simulink model "bnbRL_Plant"  (R2026a)
settings: Solver=VariableStepAuto
values from neighbouring files (symbols this model uses):
  d = 0.016    [bnbInit.m]    (also in bnbRL_Animation.m)
  g = 9.81    [bnbInit.m]
  K_BB = (R^2 * m * g * d) / (L * (m * R^2 + J))    (= 0.424676496462)    [bnbInit.m]
  L = 0.264    [bnbInit.m]    (also in bnbRL_Animation.m)
  x0 = 0    [bnbInit.m]
  xdot0 = 0    [bnbInit.m]
settings Model: Creator=user  LastModifiedBy=user

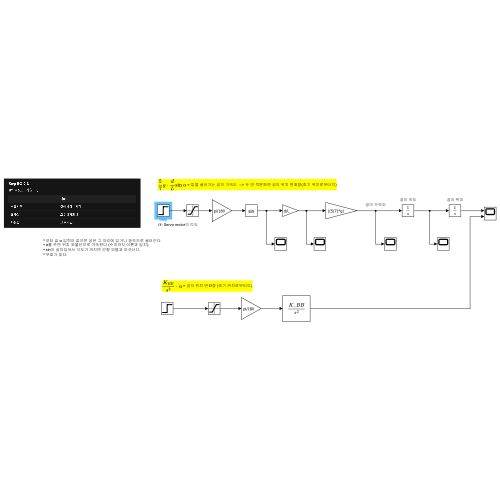
[thumbnail: Simulink's stored preview of the top-level diagram]
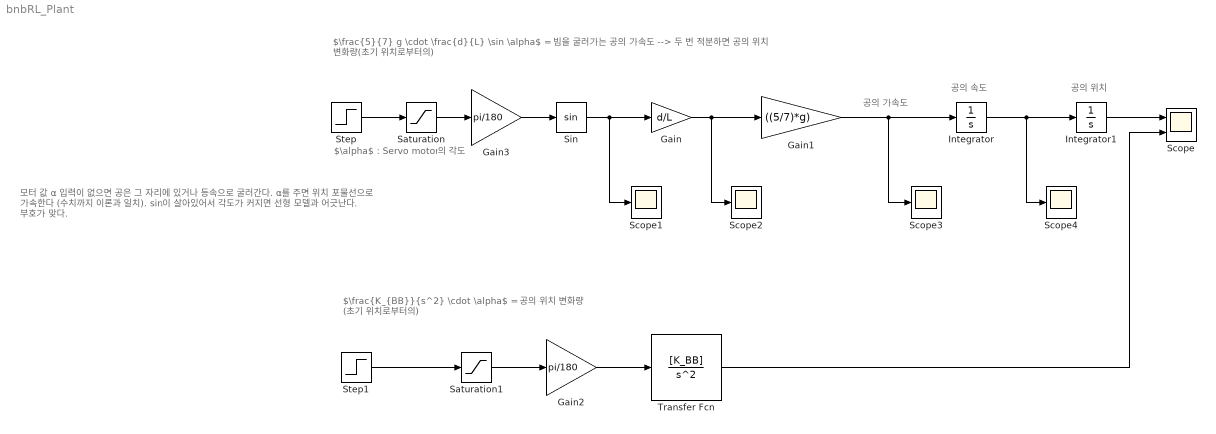
== system bnbRL_Plant ==
  note: 모터 값 α 입력이 없으면 공은 그 자리에 있거나 등속으로 굴러간다.
      | α를 주면 위치 포물선으로 가속한다 (수치까지 이론과 일치).
      | sin이 살아있어서 각도가 커지면 선형 모델과 어긋난다.
      | 부호가 맞다.
  note: 공의 가속도
  note: 공의 위치
  note: 공의 속도
  note: $\alpha$ : Servo motor의 각도
  note: $\frac{5}{7} g \cdot \frac{d}{L} \sin \alpha$ = 빔을 굴러가는 공의 가속도 --> 두 번 적분하면 공의 위치 변화량(초기 위치로부터의)
  note: $\frac{K_{BB}}{s^2} \cdot \alpha$ = 공의 위치 변화량 (초기 위치로부터의)
  Gain : Gain  Gain=d/L
  Gain1 : Gain  Gain=((5/7)*g)
  Gain2 : Gain  Gain=pi/180
  Gain3 : Gain  Gain=pi/180
  Integrator : Integrator  InitialCondition=xdot0
  Integrator1 : Integrator  InitialCondition=x0
  Saturation : Saturate  UpperLimit=90  LowerLimit=-90
  Saturation1 : Saturate  UpperLimit=90  LowerLimit=-90
  Scope : Scope  NumInputPorts=2
      settings: ActiveDisplayYMinimum=-1.0180194805194851  ActiveDisplayYMaximum=9.162175324675367
  Scope{1..4} (4 alike) : Scope
      Scope1 settings: ActiveDisplayYMinimum=-1  ActiveDisplayYMaximum=1
      Scope2 settings: ActiveDisplayYMinimum=-1  ActiveDisplayYMaximum=1  DataLoggingVariableName=ScopeData2
      Scope3 settings: ActiveDisplayYMinimum=-1  ActiveDisplayYMaximum=1  DataLoggingVariableName=ScopeData3
      Scope4 settings: ActiveDisplayYMinimum=-1  ActiveDisplayYMaximum=1  DataLoggingVariableName=ScopeData4
  Sin : Trigonometry
  Step : Step  Time=2  FinalValue=30  SampleTime=0.020
  Step1 : Step  Time=2  FinalValue=30  SampleTime=0.020
  Transfer Fcn : TransferFcn  Numerator=[K_BB]  Denominator=[1 0 0]
  wires:
  Gain1/1 -> Scope3/1, Integrator/1
  Integrator/1 -> Scope4/1, Integrator1/1
  Integrator1/1 -> Scope/1
  Step/1 -> Saturation/1
  Gain/1 -> Gain1/1, Scope2/1
  Sin/1 -> Scope1/1, Gain/1
  Step1/1 -> Saturation1/1
  Transfer Fcn/1 -> Scope/2
  Saturation/1 -> Gain3/1
  Saturation1/1 -> Gain2/1
  Gain2/1 -> Transfer Fcn/1
  Gain3/1 -> Sin/1
